simulink model "ML_UAV_3D_2"  (R2018a)
settings: Solver=ode4  StartTime=0.0  StopTime=130  FixedStep=Ts  MaxStep=2*T  MinStep=T  RelTol=1e-4
values from neighbouring files (symbols this model uses):
  Ac = 0.0331    [init_ML_UAV_3D_2.m]
  Am1_LPF = sysd.denominator{1}    [init_ML_UAV_3D_2.m]
  Am2_LPF = sysd.denominator{1}    [init_ML_UAV_3D_2.m]
  Am_coup_LPF = sysd.denominator{1}    [init_ML_UAV_3D_2.m]
  Amp_sf = 3    [init_ML_UAV_3D_2.m]
  Amp_sf_rp = 0.05*uav.m*g    [init_ML_UAV_3D_2.m]
  Bm1_LPF = sysd.numerator{1}    [init_ML_UAV_3D_2.m]
  Bm2_LPF = sysd.numerator{1}    [init_ML_UAV_3D_2.m]
  Bm_coup_LPF = sysd.numerator{1}    [init_ML_UAV_3D_2.m]
  C_S = [5;5;9]*10^-3    [init_ML_UAV_3D_2.m]
  Cd_u = 0.2    [init_ML_UAV_3D_2.m]
  dc_M_p = 6.7    [init_ML_UAV_3D_2.m]
  eps_V = 0.5    [init_ML_UAV_3D_2.m]
  g = 9.81    [init_ML_UAV_3D_2.m]
  gamma_d_p = (2*0.3/0.03*2*0.2*12/4)/10    (= 2.4)    [init_ML_UAV_3D_2.m]
  k3 = 24    [init_ML_UAV_3D_2.m]
  k4 = 0.8    [init_ML_UAV_3D_2.m]
  min_sf = 5    [init_ML_UAV_3D_2.m]
  min_sf_rp = 0.35*uav.m*g    [init_ML_UAV_3D_2.m]
  OMEGA_FILTER_OUTER = 40    [estimation.m]
  T_init = 10    [init_ML_UAV_3D_2.m]
  Tc = 1/500    (= 0.002)    [estimation.m]
  Tg = 1/ 20    (= 0.05)    [estimation.m]
  Tn = 1/500    (= 0.002)    [estimation.m]
  Ts = 1/500    (= 0.002)    [estimation.m]    (also in init_ML_UAV_3D_2.m)
  Tsc = 1/100    (= 0.01)    [estimation.m]
  Tz = 1/500    (= 0.002)    [estimation.m]
  X_GPS_offset = [0.01 0.005]    [estimation.m]
undefined symbols (not defined in the file or in its folder): Am_HPF, Am_LPF, Am_LPF2, an1, an1_v, an2, an3, Bm_HPF, Bm_LPF, Bm_LPF2, bn1, bn1_v, bn2, bn3, buoy, cable, controller, current, D_b, DiscIntNeverNeededParam, F, filters, J_u, K, kd_t, kp_t, L, Light, magnitude, MIL, Phi0, Psi0, R_b, T, Theta0, theta_q_ini, tolerences, torque_corr, uav, Vol_b, water, wave, X0_u
libraries: simulink x48, simulink_extras x10, UAV_Control x4, dspmtrx3 x2, aerolibwind2 x2
(part 2 of 6)

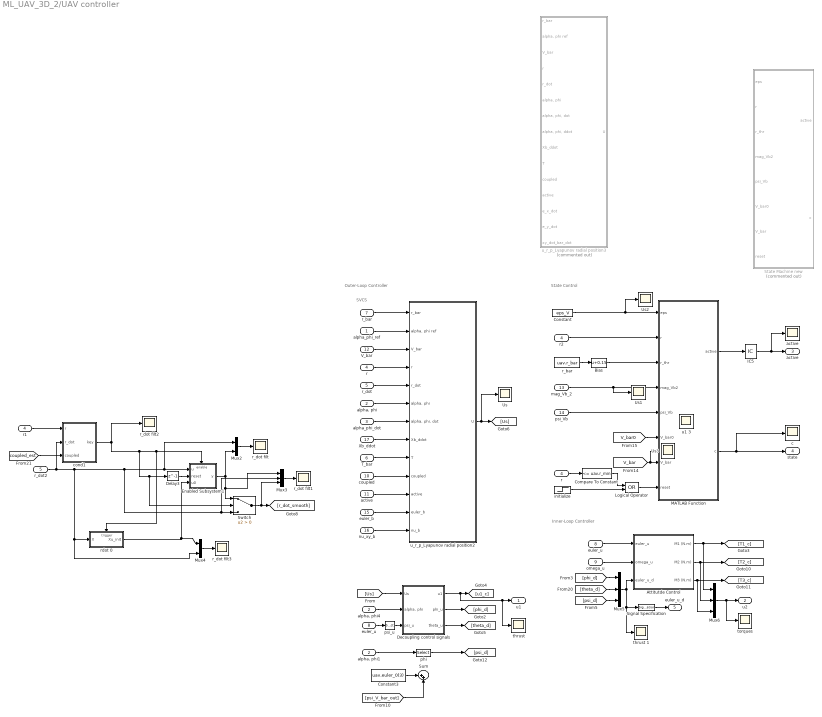
== system ML_UAV_3D_2/UAV controller ==
  note: State Control
  note: Inner-Loop Controller
  note: Outer-Loop Controller
  note: SVCS
  alpha_phi_ref : Inport
  "alpha, phi" : Inport  Port=2
  alpha_phi_dot : Inport  Port=3
  r : Inport  Port=4
  r_dot : Inport  Port=5
  T_bar : Inport  Port=6
  r_bar : Inport  Port=7
  euler_u : Inport  Port=8
  omega_u : Inport  Port=9
  coupled : Inport  Port=10
  active : Inport  Port=11
  V_bar : Inport  Port=12
  mag_Vb_2 : Inport  Port=13
  psi_Vb : Inport  Port=14
  euler_b : Inport  Port=15
  nu_xy_b : Inport  Port=16
  Xb_ddot : Inport  Port=17
  " active " : Scope
  " c " : Scope
  " phi " : Selector  InputPortWidth=2  IndexOptions=Index vector (dialog)  Indices=2  OutputSizes=1
  " r" : InportShadow  Port=4
  " r1" : InportShadow  Port=4
  Attitutde Control : Subsystem
  Bias : Bias  Bias=0.15
  Compare To Constant : simulink/Logic and Bit Operations/Compare To Constant  relop=<=  const=uav.r_min  OutDataTypeStr=boolean
  Constant : Constant  Value=eps_V
  Constant3 : Constant  Value=uav.euler_0(3)
  "Decoupling control signals " : Subsystem
  Delay3 : Delay  DelayLength=1  InitialCondition=0
  Enabled Subsystem1 : Subsystem  TreatAsAtomicUnit=on
  IC5 : InitialCondition  Value=0
  Logical Operator : Logic  Operator=OR  AllPortsSameDT=off  OutDataTypeStr=boolean
  MATLAB Function : MATLAB Function  TreatAsAtomicUnit=on
  Mux2 : Mux  Inputs=2
  Mux3 : Mux  Inputs=3
  Mux4 : Mux  Inputs=2
  Mux5 : Mux  Inputs=3
  Mux6 : Mux  Inputs=3
  Signal Specification : SignalSpecification  Dimensions=[3,1]
  State Machine new : MATLAB Function  Commented=on  TreatAsAtomicUnit=on  SystemSampleTime=Ts  mask{eps_V=0}
  Sum : Sum  Inputs=|++
  Switch : Switch  Criteria=u2 > Threshold
  Us{,1..3} (4 alike) : Scope
  "alpha, phi1" : InportShadow  Port=2
  "alpha, phi4" : InportShadow  Port=2
  cond1 : Subsystem
  "euler_u " : InportShadow  Port=8
  initialize : Step  Time=T_init  Before=1  After=0  SampleTime=0
  psi_u : Selector  InputPortWidth=3  IndexOptions=Index vector (dialog)  Indices=3  OutputSizes=1
  r2 : InportShadow  Port=4
  "r_bar " : Constant  Value=uav.r_bar
  r_dot filt{,1..3} (4 alike) : Scope
  r_dot2 : InportShadow  Port=5
  rdot 0 : Subsystem  TreatAsAtomicUnit=on
  "thrust " : Scope
  thrust 1 : Scope
  torques : Scope
  u1 3 : Scope
  u_r_p_Lyapunov radial position2 : Subsystem
  u_r_p_Lyapunov radial position3 : Subsystem  Commented=on
  u1 : Outport
  u2 : Outport  Port=2
  " active" : Outport  Port=3
  state : Outport  Port=4
  euler_u_d : Outport  Port=5
  wires:
  "Decoupling control signals "/1(u1) -> "thrust "/1, u1/1, [u1_c]
  T_bar/1 -> u_r_p_Lyapunov radial position2/9(T)
  V_bar/1 -> u_r_p_Lyapunov radial position2/3("V_bar ")
  Xb_ddot/1 -> u_r_p_Lyapunov radial position2/8(Xb_ddot)
  alpha_phi_ref/1 -> u_r_p_Lyapunov radial position2/2("alpha, phi ref")
  [V_bar0] -> MATLAB Function/6(V_bar0)
  Constant/1 -> Us2/1, MATLAB Function/1(eps)
  MATLAB Function/1(active) -> IC5/1
  MATLAB Function/2(c) -> " c "/1, state/1
  IC5/1 -> " active "/1, " active"/1
  r_bar/1 -> u_r_p_Lyapunov radial position2/1("r_bar ")
  r/1 -> Compare To Constant/1
  Compare To Constant/1 -> Logical Operator/1
  initialize/1 -> Logical Operator/2
  active/1 -> u_r_p_Lyapunov radial position2/11(active)
  "r_bar "/1 -> Bias/1
  u_r_p_Lyapunov radial position2/1(U) -> Us/1, [Us]
  Logical Operator/1 -> MATLAB Function/8(reset)
  Mux2/1 -> r_dot filt/1
  Enabled Subsystem1/1(y) -> Mux2/2, Mux3/1, Switch/1
  Switch/1 -> Mux3/3, [r_dot_smooth]
  Mux3/1 -> r_dot filt1/1
  [coupled_est] -> cond1/3(coupled)
  coupled/1 -> u_r_p_Lyapunov radial position2/10(coupled)
  r_dot2/1 -> cond1/2(r_dot), Enabled Subsystem1/1(u), Mux2/1, Mux3/2, Switch/3, rdot 0/1(X), Mux4/2
  Mux4/1 -> r_dot filt3/1
  rdot 0/1(Xu_init) -> Mux4/1, Enabled Subsystem1/3(u0)
  " r1"/1 -> cond1/1(r)
  cond1/1(key) -> Delay3/1, Switch/2, rdot 0/Trigger, Enabled Subsystem1/Enable, r_dot filt2/1
  Delay3/1 -> Enabled Subsystem1/2(reset)
  [V_bar] -> Us3/1, MATLAB Function/7(V_bar)
  Bias/1 -> MATLAB Function/3(r_thr)
  r2/1 -> MATLAB Function/2(r)
  "euler_u "/1 -> psi_u/1
  "alpha, phi4"/1 -> "Decoupling control signals "/2("alpha, phi")
  "Decoupling control signals "/3(theta_u) -> [theta_d]
  "Decoupling control signals "/2(phi_u) -> [phi_d]
  euler_u/1 -> Attitutde Control/1(euler_u)
  omega_u/1 -> Attitutde Control/2(omega_u)
  [theta_d] -> Mux5/2
  [phi_d] -> Mux5/1
  [psi_d] -> Mux5/3
  Attitutde Control/1(M1 (N.m)) -> [T1_c], Mux6/1
  Attitutde Control/2(M2 (N.m)) -> [T2_c], Mux6/2
  Attitutde Control/3(M3 (N.m)) -> [T3_c], Mux6/3
  Mux6/1 -> torques/1, u2/1
  "alpha, phi"/1 -> u_r_p_Lyapunov radial position2/6("alpha, phi")
  alpha_phi_dot/1 -> u_r_p_Lyapunov radial position2/7("alpha, phi, dot")
  " r"/1 -> u_r_p_Lyapunov radial position2/4(r)
  r_dot/1 -> u_r_p_Lyapunov radial position2/5(r_dot)
  [Us] -> "Decoupling control signals "/1(Us)
  mag_Vb_2/1 -> Us1/1, MATLAB Function/4(mag_Vb2)
  psi_Vb/1 -> MATLAB Function/5(psi_Vb)
  " phi "/1 -> [psi_d]
  "alpha, phi1"/1 -> " phi "/1
  Mux5/1 -> Signal Specification/1, thrust 1/1, Attitutde Control/3(euler_u_d)
  psi_u/1 -> "Decoupling control signals "/3(psi_u)
  Signal Specification/1 -> euler_u_d/1
  Constant3/1 -> Sum/1
  [psi_V_bar_out] -> Sum/2
  euler_b/1 -> u_r_p_Lyapunov radial position2/12(euler_b)
  nu_xy_b/1 -> u_r_p_Lyapunov radial position2/13(nu_b)

== system ML_UAV_3D_2/Wind model ==
  Bias : Bias  Bias=0.05
  Discrete Wind Gust Model : aerolibwind2/Discrete Wind Gust Model  units=Metric (MKS)  Gx=on  Gy=off  Gz=off  t_0=1  d_m=[1 1 80]  v_m=air.V_wind
      settings: SourceProductName=Aerospace Blockset
  Dryden Wind Turbulence Model (Continuous (+q +r)) : aerolibwind2/Dryden Wind Turbulence Model  (Continuous (+q -r))  Commented=on  units=Metric (MKS)  spec=MIL-F-8785C  model=Continuous Dryden (+q +r)  W20=20  Wdeg=30  TurbProb=10^-2 - Light  L_high=533.4  Wingspan=1.5  ts=0.02  Seed=[11341 23342 13423 13344]  T_on=on
      settings: SourceProductName=Aerospace Blockset
  From25 : From  Commented=on  GotoTag=X_u  TagVisibility=global
  From3 : From  Commented=on  GotoTag=DCM_b2e  TagVisibility=global
  Gain : Gain  Commented=on
  Math Function1 : Math  Commented=on  Operator=transpose  SaturateOnIntegerOverflow=on
  N3 : Scope
  Selector2 : Selector  Commented=on  InputPortWidth=3  IndexOptions=Index vector (dialog)  Indices=2  OutputSizes=1
  Selector6 : Selector  Commented=on  InputPortWidth=2  IndexOptions=Index vector (dialog)  Indices=2  OutputSizes=1
  Zero-Order Hold : ZeroOrderHold  SampleTime=-1
  magnitude : Subsystem
  V_wind : Outport
  omega_wind : Outport  Port=2
  wires:
  Selector6/1 -> Gain/1
  Gain/1 -> Dryden Wind Turbulence Model (Continuous (+q +r))/1
  Bias/1 -> Dryden Wind Turbulence Model (Continuous (+q +r))/2, Discrete Wind Gust Model/1
  Math Function1/1 -> Dryden Wind Turbulence Model (Continuous (+q +r))/3
  From3/1 -> Math Function1/1
  Dryden Wind Turbulence Model (Continuous (+q +r))/2 -> Selector2/1
  magnitude/1(Out1) -> Bias/1
  From25/1 -> Selector6/1
  [Xdot_u] -> magnitude/1(In1)
  Discrete Wind Gust Model/1 -> Zero-Order Hold/1
  Selector2/1 -> omega_wind/1
  Zero-Order Hold/1 -> V_wind/1, N3/1

== system ML_UAV_3D_2/Preprocessing Unit/smooth lower bound1 ==
  u : Inport
  Manual Switch : ManualSwitch
  Mux3 : Mux  Inputs=2
  Saturation1 : Saturate  UpperLimit=inf  LowerLimit=min_sf
  apply for lower bound only : Switch  Criteria=u2 > Threshold  Threshold=Amp_sf+min_sf
  sat : Scope
  saturation function : Fcn  Expr=Amp_sf*tanh((u(1)-(Amp_sf+min_sf))/(Amp_sf)) + (Amp_sf+min_sf)
  sat(u) : Outport
  wires:
  apply for lower bound only/1 -> Manual Switch/1
  Mux3/1 -> sat/1
  saturation function/1 -> Mux3/2, apply for lower bound only/3
  u/1 -> Saturation1/1, apply for lower bound only/1, Mux3/1, apply for lower bound only/2, saturation function/1
  Saturation1/1 -> Manual Switch/2
  Manual Switch/1 -> sat(u)/1

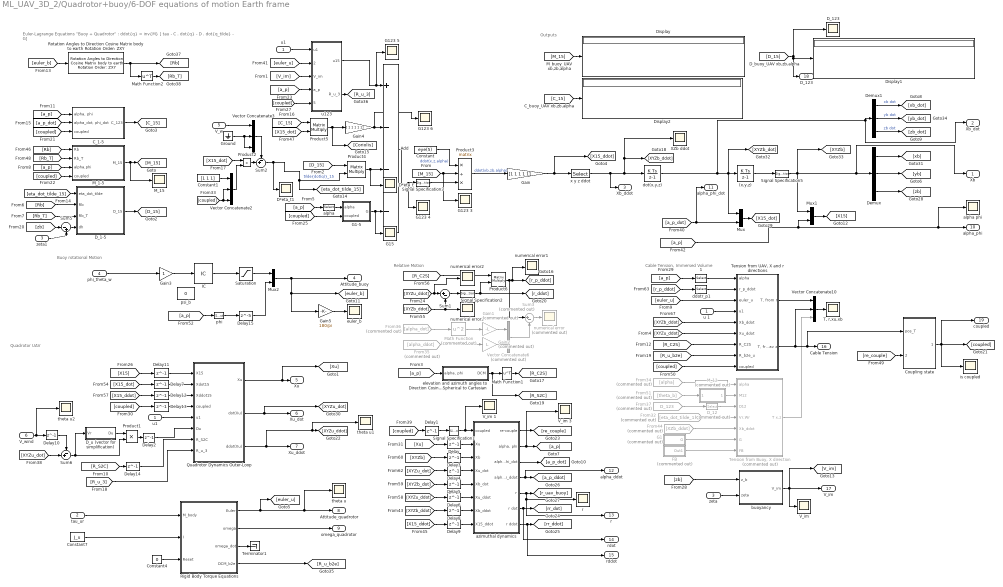
== system ML_UAV_3D_2/Quadrotor+buoy/6-DOF equations of motion Earth frame ==
  note: Relative Motion
  note: Outputs
  note: Buoy rotational Motion
  note: Cable Tension, Immersed Volume
  note: Quadrotor UAV
  note: Euler-Lagrange Equations "Buoy + Quadrotor" : ddot{q} = inv{M} [ tau - C . dot{q} - D . dot{q_tilde} - G]
  u1 : Inport
  tau_ur : Inport  Port=2
  zeta : Inport  Port=3
  phi_theta_w : Inport  Port=4
  V_w : Inport  Port=5
  V_wind : Inport  Port=6
  "  r   " : Scope
  " 1 " : Selector  InputPortWidth=2  IndexOptions=Index vector (dialog)  Indices=1  OutputSizes=2
  " alpha " : Selector  InputPortWidth=2  IndexOptions=Index vector (dialog)  Indices=1  OutputSizes=1
  (x,y,z) : DiscreteIntegrator  InitialCondition=[pos_b_ini]  SampleTime=-1  ICPrevOutput=DiscIntNeverNeededParam  ICPrevScaledInput=DiscIntNeverNeededParam
  Add : Sum  Inputs=+---
  C_1-5 : Subsystem
  Constant : Constant  Value=eye(5)
  Constant1 : Constant  Value=[1 1 1]
  Constant4 : Constant  Value=0
  Constant7 : Constant  Value=J_u
  Coupling state : Subsystem
  D*eta_t : Scope
  D*eta_t1 : Scope
  D_1-5 : Subsystem
  D_12 : Selector  Commented=on  NumberOfDimensions=2  InputPortWidth=3  IndexOptions=Starting index (dialog),Starting index (dialog)  Indices=1,1  OutputSizes=2,2
  "D_123   " : Scope
  D_u (vector for simplification) : Subsystem
  Delay{,3..9,11..14} (12 alike) : Delay  DelayLength=1
  Delay1 : Delay  DelayLength=1  InitialCondition=0
  Delay10 : Delay  DelayLength=1  InitialCondition=[0;0;0]
  Delay15 : Delay  DelayLength=5
  Delay2 : Delay  DelayLength=1  InitialCondition=[0; 0; 0]
  Demux : Demux  Outputs=3
  Demux1 : Demux  Outputs=3
  Display : Display
  Display1 : Display
  Display2 : Display
  FB : Subsystem  Commented=on
  From32 : From  Commented=on  GotoTag=eta_dot_tilde_12
  From34 : From  Commented=on  GotoTag=alpha
  From35 : From  Commented=on  GotoTag=alpha_ddot
  From36 : From  Commented=on  GotoTag=alpha_dot
  From37 : From  Commented=on  GotoTag=D_123
  From44 : From  Commented=on  GotoTag=XZb_ddot
  From51 : From  Commented=on  GotoTag=theta_b
  G1 : Subsystem  Commented=on
  G1-5 : Subsystem
  G123 {3..6} (4 alike) : Scope
  "G15 " : Scope
  Gain : Gain  Gain=[1 1 1 1 1]
  Gain1 : Gain  Commented=on  Gain=-L
  Gain2 : Gain  Commented=on  Gain=L
  Gain3 : Gain
  Gain4 : Gain  Gain=[ 1 1 1 1 1]
  Gain5 : Gain  Gain=180/pi
  Ground : Ground
  IC : InitialCondition  Value=[0 0]
  M_1-5 : Subsystem
  M_12 : Subsystem  Commented=on
  M_15 : Scope
  Math Function : Math  Commented=on  Operator=square  SaturateOnIntegerOverflow=on
  Math Function1 : Math  Operator=transpose  SaturateOnIntegerOverflow=on
  Math Function2 : Math  Operator=transpose  SaturateOnIntegerOverflow=on
  Mux : Mux  Inputs=2
  Mux1 : Mux  Inputs=2
  Mux2 : Mux  Inputs=2
  Product1 : Product  Inputs=**  SaturateOnIntegerOverflow=on  InputSameDT=on  OutDataTypeStr=Inherit: Same as first input
  Product2 : Product  Inputs=**  SaturateOnIntegerOverflow=on  InputSameDT=on  OutDataTypeStr=Inherit: Same as first input
  Product3 : Product  Inputs=*/*  Multiplication=Matrix(*)  SaturateOnIntegerOverflow=on  InputSameDT=on  OutDataTypeStr=Inherit: Same as first input
  Product4 : Product  Inputs=**  Multiplication=Matrix(*)  SaturateOnIntegerOverflow=on  InputSameDT=on  OutDataTypeStr=Inherit: Same as first input
  Product5 : Product  Inputs=**  Multiplication=Matrix(*)  SaturateOnIntegerOverflow=on  InputSameDT=on  OutDataTypeStr=Inherit: Same as first input
  Product6 : Product  Multiplication=Matrix(*)
  Quadrotor Dynamics Outer-Loop : Subsystem
  "Rigid Body Torque Equations " : Subsystem  AncestorBlock=UAV_Control/Rigid Body Torque Equations  mask(Rotational motion of rigid body){euler0=euler_u_ini, omega0=omega_u_ini}
      mask prompts: euler0 "Initial euler angles:"; omega0 "Initial angular velocites:"
      mask help: Determines the rotational motion of a 6DOF rigid body.
      mask Help:
      | alpha=Mb/I - omega x (I.omega)
      | omega_dot=alpha
      | 
      | Euler_dot=R x omega
      mask Display:
      | port_label('input',1,'M_b (N.m)','texmode','on')
      | port_label('input',2,'I (kg/m^2)','texmode','on')
      | port_label('input',3,'Reset','texmode','on')
      | 
      | port_label('output',1,'\phi,\theta,\psi (rad)','texmode','on')
      | port_label('output',2,'\omega (rad/s)','texmode','on')
      | port_label('output',3,'\alpha (rad/s^2)','texmode','on')
      | port_label('output',4,'DCM_{b2e}','texmode','on')
  Rotation Angles to Direction Cosine Matrix body to earth Rotation Order: ZXY : UAV_Control/Rotation Angles to Direction Cosine Matrix body to earth Rotation Order: ZXY
      settings: SourceProductName=UAV_Control
  Saturation : Saturate  UpperLimit=[0.15 0.15]  LowerLimit=[-0.15 -0.15]
  Signal Specification1 : SignalSpecification  Dimensions=1
  Signal Specification2 : SignalSpecification  Dimensions=3
  Signal Specification3 : SignalSpecification  Dimensions=5
  Signal Specification5 : SignalSpecification  Dimensions=3
  Sum1 : Sum  Inputs=|+-
  Sum2 : Sum  Inputs=-+|  SaturateOnIntegerOverflow=on
  Sum3 : Sum  Commented=on  Inputs=|+-
  Sum5 : Sum  Inputs=|-+  SaturateOnIntegerOverflow=on
  Sum6 : Sum  Inputs=-+|  SaturateOnIntegerOverflow=on
  "T, r,xu,xb" : Scope
  "Tension from Buoy, X direction" : Subsystem  Commented=on
  "Tension from UAV, X and r directions" : Subsystem
  Terminator1 : Terminator
  "V_im " : Scope
  V_im 1 : Scope
  V_im 3 : Scope
  Vector Concatenate10 : Concatenate  NumInputs=3
  Vector Concatenate2 : Concatenate  NumInputs=3
  Vector Concatenate3 : Concatenate  NumInputs=3
  Vector Concatenate6 : Concatenate  Commented=on
  "XZb ddot " : Scope
  "alpha phi   " : Scope
  azimuthal dynamics : Subsystem
  buoyancy : Subsystem
  ddotr_p1 : Selector  InputPortWidth=3  IndexOptions=Index vector (dialog)  Indices=1  OutputSizes=2
  dot(x,y,z) : DiscreteIntegrator  InitialCondition=[v_b_ini]  SampleTime=-1  ICPrevOutput=DiscIntNeverNeededParam  ICPrevScaledInput=DiscIntNeverNeededParam
  elevation and azimuth angles to Direction Cosine Matrix Spherical to Cartesian : Subsystem
      mask Display:
      | port_label('input',1,'\alpha, \phi','texmode','on')
      | port_label('output',1,'DCM_{S2C}','texmode','on')
  euler_b : Scope
  "is coupled " : Scope
  numerical error : Scope  Commented=on
  numerical error1 : Scope
  numerical error2 : Scope
  numerical error3 : Scope
  "phi  " : Selector  InputPortWidth=2  IndexOptions=Index vector (dialog)  Indices=2  OutputSizes=1
  psi_b : Constant  Value=0
  theta u : Scope
  theta u1 : Scope
  theta u2 : Scope
  u 1 : InportShadow
  "u1  " : InportShadow
  u123 : Subsystem
  x y z ddot : Selector  InputPortWidth=5  IndexOptions=Index vector (dialog)  Indices=[1 2 3]  OutputSizes=1
  zeta1 : InportShadow  Port=3
  Xb : Outport  Unit=m  InitialOutput=0
  Xb_dot : Outport  Port=2  Unit=m  InitialOutput=0
  Xb_ddot : Outport  Port=3  Unit=m  InitialOutput=0
  Attitude_buoy : Outport  Port=4  Unit=rad/s^2  InitialOutput=0
  Xu : Outport  Port=5  Unit=m  InitialOutput=0
  Xu_dot : Outport  Port=6  Unit=m/s  InitialOutput=0
  Xu_ddot : Outport  Port=7  Unit=m/s  InitialOutput=0
  Attitude_quadrotor : Outport  Port=8  Unit=rad  InitialOutput=0
  omega_quadrotor : Outport  Port=9  Unit=rad/s  InitialOutput=0
  alpha_phi : Outport  Port=10  Unit=m  InitialOutput=0
  alpha_phi_dot : Outport  Port=11  Unit=m  InitialOutput=0
  alpha_ddot : Outport  Port=12  Unit=m  InitialOutput=0
  "  r" : Outport  Port=13  Unit=m  InitialOutput=0
  "  rdot" : Outport  Port=14  Unit=m  InitialOutput=0
  "  rddot" : Outport  Port=15  Unit=m  InitialOutput=0
  Cable Tension : Outport  Port=16  Unit=rad/s^2  InitialOutput=0
  V_im : Outport  Port=17  Unit=m  InitialOutput=0
  "D_123 " : Outport  Port=18  Unit=m  InitialOutput=0
  coupled : Outport  Port=19  Unit=m  InitialOutput=0
  wires:
  u123/1(u15) -> G123 5/1, Add/1
  Product4/1 -> D*eta_t/1, Add/3
  [D_15] -> Product4/1
  Sum2/1 -> D*eta_t1/1, [eta_dot_tilde_15], Product4/2  "tilde{dot(q)}_15"
  G1-5/1(G) -> "G15 "/1, Add/4
  [a_p] -> Mux1/2, "alpha phi   "/1, alpha_phi/1
  [Rb] -> D_1-5/2(Rb)
  D_1-5/1(D_15) -> [D_15]
  [Rb] -> M_1-5/1(Rb)
  [a_p] -> M_1-5/3(alpha,phi)
  Demux1/3 -> [zb_dot]  "zb dot"
  Demux1/1 -> [xb_dot]  "xb dot"
  Vector Concatenate3/1 -> Sum2/1
  phi_theta_w/1 -> Gain3/1
  "Rigid Body Torque Equations "/1("Euler ") -> [euler_u], theta u/1, Attitude_quadrotor/1
  Constant7/1 -> "Rigid Body Torque Equations "/2(I)
  tau_ur/1 -> "Rigid Body Torque Equations "/1(M_body)
  [euler_u] -> u123/2(euler_u)
  [V_im] -> u123/3(V_im)
  [a_p] -> " alpha "/1
  Demux/1 -> [xb]
  Demux/2 -> [yb]
  M_1-5/1(M_15) -> M_15/1, [M_15]
  [M_15] -> G123 3/1, Product3/2
  Constant/1 -> Product3/1  "ddot(x,z,alpha)"
  Product3/1 -> Gain/1  "ddot(xb,zb,alpha)"
  IC/1 -> Saturation/1
  [a_p] -> C_1-5/1("alpha, phi ")
  [a_p_dot] -> C_1-5/2("alpha_dot, phi_dot")
  C_1-5/1(C_123) -> [C_15]
  [C_15] -> Product5/1
  Product5/1 -> [Coriolis], Gain4/1
  Gain/1 -> [X15_ddot], x y z ddot/1
  [a_p] -> u123/4(a_p)
  [r_p_ddot] -> ddotr_p1/1
  [euler_u] -> "Tension from UAV, X and r directions"/3(euler_u)
  u 1/1 -> "Tension from UAV, X and r directions"/4(u1)
  [D_15] -> Display1/1, "D_123 "/1, "D_123   "/1
  [M_15] -> Display/1
  [C_15] -> Display2/1
  (x,y,z)/1 -> Signal Specification5/1
  [zb] -> buoyancy/1(z_b)
  zeta/1 -> buoyancy/2(zeta)
  From34/1 -> "Tension from Buoy, X direction"/1(alpha)
  D_12/1 -> "Tension from Buoy, X direction"/3(D12)
  buoyancy/1(V_im) -> "V_im "/1, V_im/1, [V_im]
  M_12/1(M_12) -> "Tension from Buoy, X direction"/2(M12)
  From37/1 -> D_12/1
  From44/1 -> "Tension from Buoy, X direction"/5(Xb_ddot)
  From32/1 -> "Tension from Buoy, X direction"/4(Vr,Wr)
  [XYZb_ddot] -> "Tension from UAV, X and r directions"/5(Xb_ddot)
  G1/1(G) -> "Tension from Buoy, X direction"/6(G)
  From51/1 -> M_12/1(theta)
  x y z ddot/1 -> Xb_ddot/1, [XYZb_ddot], "XZb ddot "/1, dot(x,y,z)/1
  ddotr_p1/1 -> "Tension from UAV, X and r directions"/2(r_p_ddot)
  [XYZu_ddot] -> "Tension from UAV, X and r directions"/6(Xu_ddot)
  FB/1(Out1) -> "Tension from Buoy, X direction"/7(FB)
  Vector Concatenate10/1 -> "T, r,xu,xb"/1
  "Tension from Buoy, X direction"/1(T x,z) -> Vector Concatenate10/3
  Gain2/1 -> Vector Concatenate6/2
  [R_C2S] -> Product6/1
  Vector Concatenate6/1 -> Sum3/2
  elevation and azimuth angles to Direction Cosine Matrix Spherical to Cartesian/1(DCM) -> [R_S2C], Math Function1/1
  Product6/1 -> Sum3/1, numerical error1/1, [r_p_ddot]
  Gain1/1 -> Vector Concatenate6/1
  Math Function/1 -> Gain1/1
  Sum1/1 -> Signal Specification2/1
  [XYZu_ddot] -> numerical error2/1, Sum1/1
  Math Function1/1 -> [R_C2S]
  Sum3/1 -> numerical error/1
  [XYZb_ddot] -> numerical error3/1, Sum1/2
  From36/1 -> Math Function/1
  Mux2/1 -> Gain5/1, [euler_b], Attitude_buoy/1
  Add/1 -> Signal Specification3/1, G123 4/1
  Gain3/1 -> IC/1
  Gain4/1 -> Add/2, G123 6/1
  [eta_dot_tilde_15] -> D_1-5/1(eta_dot_tilde)
  Sum5/1 -> D_1-5/4(dh)
  [zb] -> Sum5/1
  zeta1/1 -> Sum5/2
  [coupled] -> C_1-5/3(coupled)
  [coupled] -> M_1-5/4(coupled)
  [coupled] -> G1-5/2(coupled)
  u1/1 -> u123/1(u1)
  [X15_dot] -> Product5/2
  Signal Specification2/1 -> Product6/2, [r_ddot]
  Signal Specification3/1 -> Product3/3
  Quadrotor Dynamics Outer-Loop/1(Xu) -> [Xu], Xu/1
  [coupled] -> Delay13/1
  "u1  "/1 -> Quadrotor Dynamics Outer-Loop/5(u1)
  Quadrotor Dynamics Outer-Loop/2(dot(Xu)) -> [XYZu_dot], Xu_dot/1
  [coupled] -> u123/5(coupled)
  Vector Concatenate2/1 -> Product2/2
  [Xu] -> Delay/1
  azimuthal dynamics/1(re-couple) -> [re_couple]
  azimuthal dynamics/2("alpha, phi") -> V_im 3/1, [a_p]
  azimuthal dynamics/3("alpha_dot, phi_dot ") -> [a_p_dot]
  azimuthal dynamics/4("alpha_ddot, phi_ddot") -> alpha_ddot/1, [a_p_ddot]
  Delay/1 -> azimuthal dynamics/2(Xu)
  azimuthal dynamics/5("r ") -> "  r"/1, "  r   "/1, [r_uav_buoy]
  [X15] -> Delay11/1
  Delay3/1 -> azimuthal dynamics/3(Xb)
  [X15_ddot] -> Delay12/1
  [X15_dot] -> Delay7/1
  dot(x,y,z)/1 -> Mux/1, (x,y,z)/1, [XYZb_dot], Xb_dot/1, Demux1/1
  [a_p_dot] -> alpha_phi_dot/1, Mux/2
  Mux/1 -> [X15_dot]
  Mux1/1 -> [X15]
  Signal Specification5/1 -> [XYZb], Mux1/1, Xb/1, Demux/1
  [a_p] -> " 1 "/1
  [XYZb] -> Delay3/1
  [XYZu_dot] -> Delay4/1
  [XYZb_dot] -> Delay5/1
  [XYZu_ddot] -> Delay6/1
  [XYZb_ddot] -> Delay8/1
  From35/1 -> Gain2/1
  Delay4/1 -> azimuthal dynamics/4("Xu_dot ")
  [X15_ddot] -> Delay9/1
  Delay5/1 -> azimuthal dynamics/5(Xb_dot)
  Delay6/1 -> azimuthal dynamics/6(Xu_ddot)
  Delay8/1 -> azimuthal dynamics/7("Xb_ddot   ")
  Delay9/1 -> azimuthal dynamics/8("X15_ddot  ")
  [coupled] -> Delay1/1
  Delay11/1 -> Quadrotor Dynamics Outer-Loop/1(X15)
  Delay12/1 -> Quadrotor Dynamics Outer-Loop/3(Xddot15)
  Delay7/1 -> Quadrotor Dynamics Outer-Loop/2(Xdot15)
  Delay13/1 -> Quadrotor Dynamics Outer-Loop/4(coupled)
  azimuthal dynamics/6(r dot) -> "  rdot"/1, [rr_dot]
  azimuthal dynamics/7(r ddot) -> "  rddot"/1, [rr_ddot]
  "Tension from UAV, X and r directions"/2("T, from uav z") -> Vector Concatenate10/2, Coupling state/1(pos_T), Cable Tension/1
  [re_couple] -> Coupling state/2(re_couple)
  Coupling state/1(is coupled) -> "is coupled "/1, coupled/1, [coupled]
  Quadrotor Dynamics Outer-Loop/3(ddot(Xu)) -> Xu_ddot/1, theta u1/1, [XYZu_ddot]
  "Tension from UAV, X and r directions"/1("T, from r") -> Vector Concatenate10/1
  D_u (vector for simplification)/1(Du) -> Product1/1
  [XYZu_dot] -> Sum6/2
  Sum6/1 -> D_u (vector for simplification)/1(Vr), Product1/2
  Ground/1 -> Vector Concatenate3/3, Vector Concatenate3/2
  V_w/1 -> Vector Concatenate3/1
  Product2/1 -> Sum2/2
  [X15_dot] -> Product2/1
  [coupled] -> Vector Concatenate2/2, Vector Concatenate2/3
  Constant1/1 -> Vector Concatenate2/1
  " alpha "/1 -> G1-5/1(alpha)
  Demux1/2 -> [yb_dot]  "yb dot"
  Demux/3 -> [zb]
  Gain5/1 -> euler_b/1
  [a_p] -> elevation and azimuth angles to Direction Cosine Matrix Spherical to Cartesian/1("alpha, phi")
  [R_C2S] -> "Tension from UAV, X and r directions"/7(R_C2S)
  Constant4/1 -> "Rigid Body Torque Equations "/3(Reset)
  "Rigid Body Torque Equations "/2(omega) -> omega_quadrotor/1
  "Rigid Body Torque Equations "/4(DCM_b2e) -> [R_u_b2e]
  "Rigid Body Torque Equations "/3(omega_dot) -> Terminator1/1
  [a_p] -> "phi  "/1
  Saturation/1 -> Mux2/1
  [R_S2C] -> Delay14/1
  Delay14/1 -> Quadrotor Dynamics Outer-Loop/7(R_S2C)
  u123/2(R_u_3) -> [R_u_3]
  [R_u_3] -> Quadrotor Dynamics Outer-Loop/8(R_u_3)
  [R_u_b2e] -> "Tension from UAV, X and r directions"/8("R_b2e_u ")
  " 1 "/1 -> "Tension from UAV, X and r directions"/1(alpha)
  [euler_b] -> Rotation Angles to Direction Cosine Matrix body to earth Rotation Order: ZXY/1
  Rotation Angles to Direction Cosine Matrix body to earth Rotation Order: ZXY/1 -> Math Function2/1, [Rb]
  Math Function2/1 -> [Rb_T]
  [Rb_T] -> M_1-5/2(Rb_T)
  [Rb_T] -> D_1-5/3(Rb_T)
  [coupled] -> "Tension from UAV, X and r directions"/9(coupled)
  Delay10/1 -> Sum6/1
  V_wind/1 -> Delay10/1, theta u2/1
  Product1/1 -> Delay2/1
  Delay2/1 -> Quadrotor Dynamics Outer-Loop/6(Du)
  Delay1/1 -> Signal Specification1/1
  Signal Specification1/1 -> V_im 1/1, azimuthal dynamics/1(coupled)
  "phi  "/1 -> Delay15/1
  Delay15/1 -> Mux2/2

== system ML_UAV_3D_2/Save to file/mean absolute error ==
  In1 : Inport
  Abs : Abs
  Add : Sum
  Constant : Constant  Value=T
  Delay : Delay  DelayLength=1
  IC : InitialCondition
  Product1 : Product  Inputs=*/
  Product2 : Product  Inputs=*/
  Out1 : Outport
  wires:
  Product2/1 -> IC/1
  Add/1 -> Product1/1, Delay/1
  Delay/1 -> Add/1
  [time] -> Product2/1
  In1/1 -> Abs/1
  Product1/1 -> Out1/1
  Constant/1 -> Product2/2
  IC/1 -> Product1/2
  Abs/1 -> Add/2

== system ML_UAV_3D_2/Scope/absolute mean ==
  u : Inport
  Abs : Abs
  Bias : Bias  Bias=1/1000
  Clock : Clock
  Current velocity : Scope
  Current velocity1 : Scope
  Current velocity2 : Scope
  Discrete-Time Integrator : DiscreteIntegrator  gainval=1  SampleTime=Ts  ICPrevOutput=DiscIntNeverNeededParam  ICPrevScaledInput=DiscIntNeverNeededParam
  Divide1 : Product  Inputs=*/
  mean : Outport
  wires:
  Discrete-Time Integrator/1 -> Current velocity1/1, Divide1/1
  Abs/1 -> Discrete-Time Integrator/1
  u/1 -> Current velocity/1, Abs/1
  Divide1/1 -> mean/1
  Clock/1 -> Bias/1
  Bias/1 -> Current velocity2/1, Divide1/2

== system ML_UAV_3D_2/Scope/absolute mean1 ==
  u : Inport
  Abs : Abs
  Bias : Bias  Bias=1/1000
  Clock : Clock
  Current velocity : Scope
  Current velocity1 : Scope
  Current velocity2 : Scope
  Discrete-Time Integrator : DiscreteIntegrator  gainval=1  SampleTime=Ts  ICPrevOutput=DiscIntNeverNeededParam  ICPrevScaledInput=DiscIntNeverNeededParam
  Divide1 : Product  Inputs=*/
  mean : Outport
  wires:
  Clock/1 -> Bias/1
  Divide1/1 -> mean/1
  u/1 -> Abs/1, Current velocity/1
  Abs/1 -> Discrete-Time Integrator/1
  Discrete-Time Integrator/1 -> Divide1/1, Current velocity1/1
  Bias/1 -> Divide1/2, Current velocity2/1

== system ML_UAV_3D_2/Sensors and Filters/Coupling detection by r ==
  In1 : Inport
  In2 : Inport  Port=2
  Constant1 : Constant  Value=0
  Coupling state : Subsystem
  Data Type Conversion : DataTypeConversion  OutDataTypeStr=double
  IC2 : InitialCondition  Value=0
  Switch14 : Switch  Criteria=u2 > Threshold  Threshold=0.5
  cable length with safety margine : simulink/Logic and Bit Operations/Compare To Constant  relop=>=  const=cable.L_0+0.005  OutDataTypeStr=boolean
  is coupled {,2..4} (4 alike) : Scope
  is coupled : Outport
  wires:
  IC2/1 -> Switch14/3
  In1/1 -> is coupled 3/1, Coupling state/1(r_est), is coupled 2/1, cable length with safety margine/1
  Switch14/1 -> [re_couple]
  cable length with safety margine/1 -> is coupled 4/1, Data Type Conversion/1
  [re_couple] -> Coupling state/2(re_couple)
  Data Type Conversion/1 -> IC2/1
  Coupling state/1(is coupled) -> is coupled/1, "is coupled "/1
  Constant1/1 -> Switch14/1
  In2/1 -> Switch14/2

== system ML_UAV_3D_2/Sensors and Filters/Data processing ==
  Acc : Inport
  "GPS " : Inport  Port=2
  p,q,r : Inport  Port=3
  Sonar : Inport  Port=4
  Estimate Attitude : Subsystem  TreatAsAtomicUnit=on  SystemSampleTime=Tc
  Estimate Position : Subsystem  TreatAsAtomicUnit=on  SystemSampleTime=Tc
  "Euler " : Selector  InputPortWidth=5  IndexOptions=Index vector (dialog)  Indices=[3]  OutputSizes=1
  GPS : InportShadow  Port=2
  Xe_est : Outport
  Ve_est : Outport  Port=2
  q_gyro : Outport  Port=3
  "q_est " : Outport  Port=4
  pitch_est : Outport  Port=5
  wires:
  GPS/1 -> "Euler "/1
  Acc/1 -> Estimate Attitude/1(Acc)
  p,q,r/1 -> Estimate Attitude/2(q)
  "Euler "/1 -> Estimate Attitude/3(Euler)
  Estimate Attitude/2(q_f) -> "q_est "/1
  "GPS "/1 -> Estimate Position/1(OptiTrack)
  Estimate Position/1(Xe) -> Xe_est/1
  Estimate Position/2(Ve) -> Ve_est/1
  Estimate Attitude/1(q_g) -> q_gyro/1
  Sonar/1 -> Estimate Position/3(Sonar)
  Estimate Attitude/3(" pitch") -> Estimate Position/2("pitch, Kalman"), pitch_est/1

== system ML_UAV_3D_2/Sensors and Filters/GPS//INS ==
  X : Inport
  X_dot : Inport  Port=2
  X_ddot : Inport  Port=3
  q : Inport  Port=4
  theta : Inport  Port=5
  Discrete Derivative1 : simulink/Discrete/Discrete Derivative  gainval=1.0  ICPrevScaledInput=0.0  OutMin=[]  OutMax=[]  OutDataType=fixdt(1, 16)  OutScaling=2^-10  DoSatur=off
  Discrete Derivative2 : simulink/Discrete/Discrete Derivative  gainval=1.0  ICPrevScaledInput=0.0  OutMin=[]  OutMax=[]  OutDataType=fixdt(1, 16)  OutScaling=2^-10  DoSatur=off
  GPS noise : RandomNumber  Variance=5/10000  Seed=123  SampleTime=Tg
  Gain : Gain  Gain=0.25
  Gain1 : Gain  Gain=0.5
  Gain2 : Gain
  Gain3 : Gain
  Gain4 : Gain
  IMU noise : RandomNumber  Variance=1/10000  Seed=2235  SampleTime=Ts
  Low Pass Filter{1,3..5} (4 alike) : DiscreteTransferFcn  Numerator=filters.Bm_LPF2  Denominator=filters.Am_LPF2
  Low Pass Filter2 : DiscreteTransferFcn  Numerator=filters.Bm_LPF  Denominator=filters.Am_LPF
  Mux4 : Mux  Inputs=3
  Rate Transition : RateTransition
  Rate Transition1 : RateTransition
  Sum{1,3..6} (5 alike) : Sum  Inputs=++|
  q1 : Scope
  q2 : Scope
  q3 : Scope
  X_est : Outport
  X_dot_est : Outport  Port=2
  q_est : Outport  Port=3
  theta_est : Outport  Port=4
  X_ddot_est : Outport  Port=5
  wires:
  Sum4/1 -> X_dot_est/1
  Low Pass Filter1/1 -> Low Pass Filter3/1
  Gain3/1 -> Sum6/1
  q/1 -> Sum6/2
  theta/1 -> Sum5/2
  Gain2/1 -> Sum5/1
  Rate Transition1/1 -> Low Pass Filter2/1
  IMU noise/1 -> Rate Transition1/1
  Mux4/1 -> Gain1/1
  X/1 -> Sum3/2
  GPS noise/1 -> Rate Transition/1
  Rate Transition/1 -> Low Pass Filter1/1
  Sum5/1 -> theta_est/1
  X_dot/1 -> Sum4/2
  Sum3/1 -> X_est/1
  Sum6/1 -> q_est/1
  Low Pass Filter2/1 -> Gain3/1, Gain2/1, q2/1
  Low Pass Filter3/1 -> Mux4/3, Mux4/2, Mux4/1
  Discrete Derivative1/1 -> Low Pass Filter4/1
  Gain1/1 -> Discrete Derivative1/1, Sum3/1, q1/1
  Gain/1 -> Discrete Derivative2/1, Sum4/1, q3/1
  Discrete Derivative2/1 -> Low Pass Filter5/1
  X_ddot/1 -> Sum1/2
  Gain4/1 -> Sum1/1
  Sum1/1 -> X_ddot_est/1
  Low Pass Filter4/1 -> Gain/1
  Low Pass Filter5/1 -> Gain4/1

== system ML_UAV_3D_2/Sensors and Filters/Sensors ==
  note: Gyro noise destroys the estimation
  note: Acc noise does not affect estimation
  "q " : Inport
  Ab : Inport  Port=2
  Xe : Inport  Port=3
  Euler : Inport  Port=4
  " Sonar (10Hz) (true elevation instead real sonar signal)" : Subsystem
  Accelerometer (500Hz) : Subsystem  TreatAsAtomicUnit=on  SystemSampleTime=Ts
  "GPS (10Hz) " : Subsystem  TreatAsAtomicUnit=on  SystemSampleTime=Tg
  Gyro (500Hz) : Subsystem  TreatAsAtomicUnit=on  SystemSampleTime=Ts
  RT : RateTransition  OutPortSampleTime=Ts
  Rate Transition : RateTransition
  Rate Transition1 : RateTransition
  Rate Transition2 : RateTransition  Deterministic=off  InitialCondition=[X0_u Theta0 1 1]
  Z : Selector  InputPortWidth=5  IndexOptions=Index vector (dialog)  Indices=2  OutputSizes=1
  acc : Scope  Commented=on
  pqr : Scope  Commented=on
  rotation matrix R : Subsystem
  Acc : Outport
  GPS : Outport  Port=2
  " q" : Outport  Port=3
  Sonar : Outport  Port=4
  wires:
  Xe/1 -> "GPS (10Hz) "/1(Xe)
  Ab/1 -> RT/1
  "q "/1 -> Gyro (500Hz)/1(q)
  Euler/1 -> rotation matrix R/1(angle (rad)), "GPS (10Hz) "/2(Euler)
  Accelerometer (500Hz)/1(Acc) -> Rate Transition1/1
  Gyro (500Hz)/1(" q") -> Rate Transition/1
  Z/1 -> " Sonar (10Hz) (true elevation instead real sonar signal)"/1(sonar (m))
  " Sonar (10Hz) (true elevation instead real sonar signal)"/1(calib sonar (m)) -> Sonar/1
  Rate Transition/1 -> pqr/1, " q"/1
  Rate Transition1/1 -> acc/1, Acc/1
  RT/1 -> Accelerometer (500Hz)/1(Ab)
  rotation matrix R/1(R) -> "GPS (10Hz) "/3(DCM_b2e)
  Rate Transition2/1 -> Z/1, GPS/1
  "GPS (10Hz) "/1(GPS) -> Rate Transition2/1

== system ML_UAV_3D_2/Sensors and Filters/Sterio camera + encoder ==
  note: the error in alpha should relate to the stereo camera accuracy and the radial distance:
      | alpha = atan( 2cm / 7 m) = 0.0029 rad.
  "alpha, phi" : Inport
  alpha_phi_dot : Inport  Port=2
  alpha_phi_ddot : Inport  Port=3
  r : Inport  Port=4
  r_dot : Inport  Port=5
  r_ddot : Inport  Port=6
  Discrete Derivative{,1..3} (4 alike) : simulink/Discrete/Discrete Derivative  gainval=1.0  ICPrevScaledInput=0.0  OutMin=[]  OutMax=[]  OutDataType=fixdt(1, 16)  OutScaling=2^-10  DoSatur=off
  Gain1 : Gain  Gain=0.5
  Gain2 : Gain  Gain=0.3
  Gain4 : Gain
  Gain5 : Gain
  Gain6 : Gain  Gain=0.25
  Gain7 : Gain  Gain=0.5
  Low Pass Filter{1..9} (9 alike) : DiscreteTransferFcn  Numerator=filters.Bm_LPF2  Denominator=filters.Am_LPF2
  Low Pass Filter10 : DiscreteTransferFcn  Commented=on  Numerator=Bm_LPF2  Denominator=Am_LPF2
  Low Pass Filter11 : DiscreteTransferFcn  Commented=on  Numerator=filters.Bm_LPF2  Denominator=filters.Am_LPF2
  Rate Transition1 : RateTransition
  Rate Transition2 : RateTransition
  Sum{1..2,7..10} (6 alike) : Sum  Inputs=++|
  stereo cam noise (location in frame) : RandomNumber  Variance=1/100000  Seed=5684  SampleTime=Tsc
  sterio cam noise (range) : RandomNumber  Variance=1/1000  Seed=1142  SampleTime=Tsc
  alpha_phi_est : Outport
  alpha_phi_dot_est : Outport  Port=2
  r_est : Outport  Port=3
  r_dot_est : Outport  Port=4
  alpha_phi_ddot_est : Outport  Port=5
  r_ddot_est : Outport  Port=6
  wires:
  Rate Transition2/1 -> Low Pass Filter3/1
  stereo cam noise (location in frame)/1 -> Rate Transition2/1
  Gain5/1 -> Sum8/1
  Sum10/1 -> r_dot_est/1
  Discrete Derivative/1 -> Low Pass Filter8/1
  alpha_phi_dot/1 -> Sum9/2
  Gain4/1 -> Sum7/1
  Discrete Derivative1/1 -> Low Pass Filter7/1
  Sum7/1 -> alpha_phi_est/1
  Sum8/1 -> r_est/1
  r/1 -> Sum8/2
  "alpha, phi"/1 -> Sum7/2
  r_dot/1 -> Sum10/2
  Sum9/1 -> alpha_phi_dot_est/1
  sterio cam noise (range)/1 -> Rate Transition1/1
  Rate Transition1/1 -> Low Pass Filter1/1
  Sum1/1 -> alpha_phi_ddot_est/1
  Discrete Derivative2/1 -> Low Pass Filter6/1
  Gain6/1 -> Discrete Derivative2/1, Sum9/1
  Gain1/1 -> Sum1/1
  alpha_phi_ddot/1 -> Sum1/2
  r_ddot/1 -> Sum2/2
  Discrete Derivative3/1 -> Low Pass Filter9/1
  Gain2/1 -> Sum2/1
  Sum2/1 -> r_ddot_est/1
  Gain7/1 -> Discrete Derivative3/1, Sum10/1
  Low Pass Filter2/1 -> Gain7/1
  Low Pass Filter4/1 -> Gain2/1
  Low Pass Filter5/1 -> Gain6/1
  Low Pass Filter6/1 -> Gain1/1
  Low Pass Filter7/1 -> Low Pass Filter5/1
  Low Pass Filter8/1 -> Low Pass Filter2/1
  Low Pass Filter9/1 -> Low Pass Filter4/1
  Low Pass Filter3/1 -> Gain4/1, Discrete Derivative1/1
  Low Pass Filter1/1 -> Gain5/1, Discrete Derivative/1

== system ML_UAV_3D_2/Sensors and Filters/quadrotor position from relative buoy-UAV position ==
  X_u : Inport
  Xdot_u : Inport  Port=2
  Xddot_u : Inport  Port=3
  r : Inport  Port=4
  r_dot : Inport  Port=5
  r_ddot : Inport  Port=6
  "alpha, phi" : Inport  Port=7
  "(alpha, phi)_dot" : Inport  Port=8
  "(alpha, phi)_ddot" : Inport  Port=9
  Buoy's States from UAV : MATLAB Function  TreatAsAtomicUnit=on
  Demux : Demux  Outputs=2
  Demux3 : Demux  Outputs=2
  Demux4 : Demux  Outputs=2
  Signal Specification{,1..8} (9 alike) : SignalSpecification  Dimensions=[3,1]
  UAV's Spherical States : MATLAB Function  TreatAsAtomicUnit=on
  theta u1 : Scope
  theta u4 : Scope
  theta u6 : Scope
  Xb : Outport
  Xdot_b : Outport  Port=2
  Xddot_b : Outport  Port=3
  wires:
  r/1 -> UAV's Spherical States/1(r)
  Xdot_u/1 -> Signal Specification5/1
  X_u/1 -> Signal Specification/1
  r_dot/1 -> UAV's Spherical States/2(r_dot)
  Buoy's States from UAV/3(rb_ddot) -> Signal Specification3/1
  Buoy's States from UAV/1(rb) -> Signal Specification1/1
  r_ddot/1 -> UAV's Spherical States/3(r_ddot)
  Xddot_u/1 -> Signal Specification2/1
  Demux/1 -> UAV's Spherical States/4(alpha)
  Demux/2 -> UAV's Spherical States/7(phi)
  "alpha, phi"/1 -> Demux/1  "alpha"
  "(alpha, phi)_dot"/1 -> Demux3/1
  Demux3/1 -> UAV's Spherical States/5(alpha_dot)
  Demux4/1 -> UAV's Spherical States/6(alpha_ddot)
  "(alpha, phi)_ddot"/1 -> Demux4/1
  Demux3/2 -> UAV's Spherical States/8(phi_dot)
  Demux4/2 -> UAV's Spherical States/9(phi_ddot)
  UAV's Spherical States/4(R_S2C) -> Buoy's States from UAV/4(R_S2C)
  UAV's Spherical States/2(br_dot) -> Signal Specification7/1
  UAV's Spherical States/1(br) -> Signal Specification6/1
  UAV's Spherical States/3(br_ddot) -> Signal Specification8/1
  Signal Specification/1 -> Buoy's States from UAV/1(ru)
  Signal Specification2/1 -> Buoy's States from UAV/3(ru_ddot)
  Signal Specification1/1 -> theta u4/1, Xb/1
  Buoy's States from UAV/2(rb_dot) -> Signal Specification4/1
  Signal Specification4/1 -> theta u6/1, Xdot_b/1
  Signal Specification5/1 -> Buoy's States from UAV/2(ru_dot)
  Signal Specification6/1 -> Buoy's States from UAV/5(br)
  Signal Specification8/1 -> Buoy's States from UAV/7(br_ddot)
  Signal Specification7/1 -> Buoy's States from UAV/6(br_dot)
  Signal Specification3/1 -> theta u1/1, Xddot_b/1

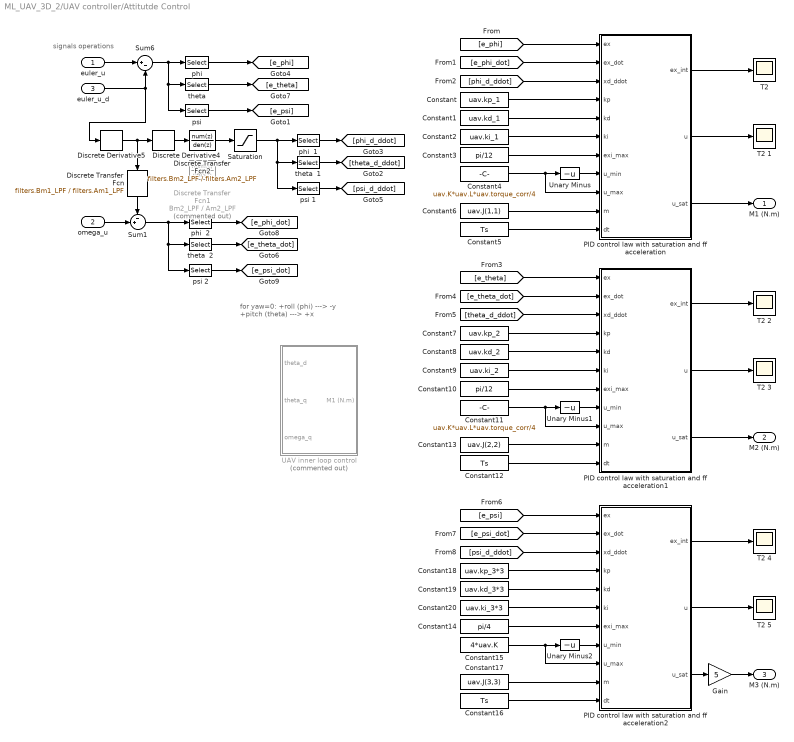
== system ML_UAV_3D_2/UAV controller/Attitutde Control ==
  note: for yaw=0:
      | +roll (phi) ---> -y
      | +pitch (theta) ---> +x
  note: signals operations
  euler_u : Inport
  omega_u : Inport  Port=2
  euler_u_d : Inport  Port=3
  "  phi  " : Selector  InputPortWidth=3  IndexOptions=Index vector (dialog)  Indices=1  OutputSizes=1
  "  phi  1" : Selector  InputPortWidth=3  IndexOptions=Index vector (dialog)  Indices=1  OutputSizes=1
  "  phi  2" : Selector  InputPortWidth=3  IndexOptions=Index vector (dialog)  Indices=1  OutputSizes=1
  "  theta  " : Selector  InputPortWidth=3  IndexOptions=Index vector (dialog)  Indices=2  OutputSizes=1
  "  theta  1" : Selector  InputPortWidth=3  IndexOptions=Index vector (dialog)  Indices=2  OutputSizes=1
  "  theta  2" : Selector  InputPortWidth=3  IndexOptions=Index vector (dialog)  Indices=2  OutputSizes=1
  " psi " : Selector  InputPortWidth=3  IndexOptions=Index vector (dialog)  Indices=3  OutputSizes=1
  " psi 1" : Selector  InputPortWidth=3  IndexOptions=Index vector (dialog)  Indices=3  OutputSizes=1
  " psi 2" : Selector  InputPortWidth=3  IndexOptions=Index vector (dialog)  Indices=3  OutputSizes=1
  Constant : Constant  Value=uav.kp_1
  Constant1 : Constant  Value=uav.kd_1
  Constant10 : Constant  Value=pi/12
  Constant11 : Constant  Value=uav.K*uav.L*uav.torque_corr/4
  Constant12 : Constant  Value=Ts
  Constant13 : Constant  Value=uav.J(2,2)
  Constant14 : Constant  Value=pi/4
  Constant15 : Constant  Value=4*uav.K
  Constant16 : Constant  Value=Ts
  Constant17 : Constant  Value=uav.J(3,3)
  Constant18 : Constant  Value=uav.kp_3*3
  Constant19 : Constant  Value=uav.kd_3*3
  Constant2 : Constant  Value=uav.ki_1
  Constant20 : Constant  Value=uav.ki_3*3
  Constant3 : Constant  Value=pi/12
  Constant4 : Constant  Value=uav.K*uav.L*uav.torque_corr/4
  Constant5 : Constant  Value=Ts
  Constant6 : Constant  Value=uav.J(1,1)
  Constant7 : Constant  Value=uav.kp_2
  Constant8 : Constant  Value=uav.kd_2
  Constant9 : Constant  Value=uav.ki_2
  Discrete Transfer Fcn : DiscreteTransferFcn  Numerator=filters.Bm1_LPF  Denominator=filters.Am1_LPF  InitialStates=[0;0;0]
  Discrete Transfer Fcn1 : DiscreteTransferFcn  Commented=on  Numerator=Bm2_LPF  Denominator=Am2_LPF  InitialStates=[0 0 0]
  Discrete Transfer Fcn2 : DiscreteTransferFcn  Numerator=filters.Bm2_LPF  Denominator=filters.Am2_LPF
  Discrete Derivative4 : simulink/Discrete/Discrete Derivative  gainval=1.0  ICPrevScaledInput=uav.euler_0  OutMin=[]  OutMax=[]  OutDataType=fixdt(1, 16)  OutScaling=2^-10  DoSatur=off
  Discrete Derivative5 : simulink/Discrete/Discrete Derivative  gainval=1.0  ICPrevScaledInput=[uav.euler_0]/Ts  OutMin=[]  OutMax=[]  OutDataType=fixdt(1, 16)  OutScaling=2^-10  DoSatur=off
  Gain : Gain  Gain=5
  PID control law with saturation and ff acceleration : MATLAB Function  TreatAsAtomicUnit=on
  PID control law with saturation and ff acceleration1 : MATLAB Function  TreatAsAtomicUnit=on
  PID control law with saturation and ff acceleration2 : MATLAB Function  TreatAsAtomicUnit=on
  Saturation : Saturate  UpperLimit=[5 5 5]  LowerLimit=-[5 5 5]
  Sum1 : Sum  Inputs=-+|
  Sum6 : Sum  Inputs=|+-
  T2 {,1..5} (6 alike) : Scope
  UAV inner loop control : Subsystem  Commented=on
  Unary Minus : UnaryMinus
  Unary Minus1 : UnaryMinus
  Unary Minus2 : UnaryMinus
  M1 (N.m) : Outport
  M2 (N.m) : Outport  Port=2
  M3 (N.m) : Outport  Port=3
  wires:
  "  phi  "/1 -> [e_phi]
  omega_u/1 -> Sum1/2
  "  theta  "/1 -> [e_theta]
  euler_u_d/1 -> Discrete Derivative5/1, Sum6/2
  Discrete Derivative5/1 -> Discrete Derivative4/1, Discrete Transfer Fcn/1
  Sum6/1 -> " psi "/1, "  theta  "/1, "  phi  "/1
  euler_u/1 -> Sum6/1
  Sum1/1 -> " psi 2"/1, "  theta  2"/1, "  phi  2"/1
  " psi "/1 -> [e_psi]
  Saturation/1 -> "  phi  1"/1, " psi 1"/1, "  theta  1"/1
  "  phi  1"/1 -> [phi_d_ddot]
  "  theta  1"/1 -> [theta_d_ddot]
  " psi 1"/1 -> [psi_d_ddot]
  "  phi  2"/1 -> [e_phi_dot]
  "  theta  2"/1 -> [e_theta_dot]
  " psi 2"/1 -> [e_psi_dot]
  [e_phi_dot] -> PID control law with saturation and ff acceleration/2(ex_dot)
  [e_phi] -> PID control law with saturation and ff acceleration/1(ex)
  [phi_d_ddot] -> PID control law with saturation and ff acceleration/3(xd_ddot)
  Constant/1 -> PID control law with saturation and ff acceleration/4(kp)
  Constant2/1 -> PID control law with saturation and ff acceleration/6(ki)
  Constant1/1 -> PID control law with saturation and ff acceleration/5(kd)
  Constant3/1 -> PID control law with saturation and ff acceleration/7(exi_max)
  Constant4/1 -> PID control law with saturation and ff acceleration/9(u_max), Unary Minus/1
  Unary Minus/1 -> PID control law with saturation and ff acceleration/8(u_min)
  Constant5/1 -> PID control law with saturation and ff acceleration/11(dt)
  Constant6/1 -> PID control law with saturation and ff acceleration/10(m)
  PID control law with saturation and ff acceleration/1(ex_int) -> "T2 "/1
  PID control law with saturation and ff acceleration/2(u) -> T2 1/1
  PID control law with saturation and ff acceleration/3(u_sat) -> M1 (N.m)/1
  PID control law with saturation and ff acceleration1/2(u) -> T2 3/1
  [e_theta_dot] -> PID control law with saturation and ff acceleration1/2(ex_dot)
  Constant13/1 -> PID control law with saturation and ff acceleration1/10(m)
  [e_theta] -> PID control law with saturation and ff acceleration1/1(ex)
  [theta_d_ddot] -> PID control law with saturation and ff acceleration1/3(xd_ddot)
  PID control law with saturation and ff acceleration1/3(u_sat) -> M2 (N.m)/1
  Constant7/1 -> PID control law with saturation and ff acceleration1/4(kp)
  Constant9/1 -> PID control law with saturation and ff acceleration1/6(ki)
  Constant8/1 -> PID control law with saturation and ff acceleration1/5(kd)
  Unary Minus1/1 -> PID control law with saturation and ff acceleration1/8(u_min)
  Constant10/1 -> PID control law with saturation and ff acceleration1/7(exi_max)
  PID control law with saturation and ff acceleration1/1(ex_int) -> T2 2/1
  Constant11/1 -> PID control law with saturation and ff acceleration1/9(u_max), Unary Minus1/1
  Constant12/1 -> PID control law with saturation and ff acceleration1/11(dt)
  PID control law with saturation and ff acceleration2/3(u_sat) -> Gain/1
  Constant14/1 -> PID control law with saturation and ff acceleration2/7(exi_max)
  PID control law with saturation and ff acceleration2/1(ex_int) -> T2 4/1
  Unary Minus2/1 -> PID control law with saturation and ff acceleration2/8(u_min)
  Constant18/1 -> PID control law with saturation and ff acceleration2/4(kp)
  Constant15/1 -> PID control law with saturation and ff acceleration2/9(u_max), Unary Minus2/1
  [e_psi] -> PID control law with saturation and ff acceleration2/1(ex)
  [psi_d_ddot] -> PID control law with saturation and ff acceleration2/3(xd_ddot)
  Constant16/1 -> PID control law with saturation and ff acceleration2/11(dt)
  Constant17/1 -> PID control law with saturation and ff acceleration2/10(m)
  PID control law with saturation and ff acceleration2/2(u) -> T2 5/1
  [e_psi_dot] -> PID control law with saturation and ff acceleration2/2(ex_dot)
  Constant20/1 -> PID control law with saturation and ff acceleration2/6(ki)
  Constant19/1 -> PID control law with saturation and ff acceleration2/5(kd)
  Discrete Derivative4/1 -> Discrete Transfer Fcn2/1
  Discrete Transfer Fcn/1 -> Sum1/1
  Discrete Transfer Fcn2/1 -> Saturation/1
  Gain/1 -> M3 (N.m)/1

== system ML_UAV_3D_2/UAV controller/Decoupling control signals  ==
  Us : Inport
  "alpha, phi" : Inport  Port=2
  psi_u : Inport  Port=3
  Constant1 : Constant  Value=uav.LIMIT_uCMD_HEIGHT
  Constant2 : Constant  Value=uav.LIMIT_CMD_PITCH
  Constant3 : Constant  Value=uav.m*g*0.5
  Demux : Demux  Outputs=3
  Demux1 : Demux  Outputs=2
  U_C{,1..5} (6 alike) : Scope
  control signals decoupling : MATLAB Function  TreatAsAtomicUnit=on
  u1 : Outport
  phi_u : Outport  Port=2
  theta_u : Outport  Port=3
  wires:
  Constant3/1 -> control signals decoupling/7(uz_min)
  Constant1/1 -> control signals decoupling/8(u1_max)
  Constant2/1 -> control signals decoupling/9(tilt_max)
  Demux/2 -> control signals decoupling/2(ua)
  Demux/1 -> control signals decoupling/1(ur)
  Demux/3 -> control signals decoupling/3(uf)
  Us/1 -> U_C4/1, Demux/1
  Demux1/2 -> control signals decoupling/5(phi)
  Demux1/1 -> control signals decoupling/4(alpha)
  psi_u/1 -> control signals decoupling/6(psi_u)
  control signals decoupling/4(theta_u) -> U_C3/1, theta_u/1
  control signals decoupling/1(u_C) -> U_C/1
  control signals decoupling/2(u1) -> U_C1/1, u1/1
  control signals decoupling/3(phi_u) -> U_C2/1, phi_u/1
  "alpha, phi"/1 -> U_C5/1, Demux1/1

== system ML_UAV_3D_2/UAV controller/Enabled Subsystem1 ==
  u : Inport
  reset : Inport  Port=2
  u0 : Inport  Port=3
  Enable : EnablePort
  Logical Operator : Logic  Operator=NOT  AllPortsSameDT=off  OutDataTypeStr=boolean
  Low Pass Filter5 : DiscreteTransferFcn  Numerator=filters.Bm_rdeL_LPF  Denominator=filters.Am_rdeL_LPF  InitialStatesSource=Input port  ExternalReset=Level
      settings: InputPortMap=u0,r7,p5
  Mux2 : Mux  Inputs=2
  adjustment for this specific transfer function : Gain  Gain=84.6505602
  r_dot filt : Scope
  r_dot filt1 : Scope
  y : Outport
  wires:
  u/1 -> Mux2/2, Low Pass Filter5/1
  Low Pass Filter5/1 -> Mux2/1, y/1
  Logical Operator/1 -> r_dot filt1/1, Low Pass Filter5/2
  u0/1 -> adjustment for this specific transfer function/1
  Mux2/1 -> r_dot filt/1
  adjustment for this specific transfer function/1 -> Low Pass Filter5/3
  reset/1 -> Logical Operator/1

== system ML_UAV_3D_2/UAV controller/cond1 ==
  r : Inport
  r_dot : Inport  Port=2
  coupled : Inport  Port=3
  Constant : Constant  Value=cable.L_0
  Constant2 : Constant  Value=Ts
  MATLAB Function : MATLAB Function  TreatAsAtomicUnit=on
  r_dot filt2 : Scope
  key : Outport
  wires:
  r/1 -> MATLAB Function/1(r)
  Constant/1 -> MATLAB Function/4(Lc)
  Constant2/1 -> MATLAB Function/5(dt)
  MATLAB Function/1(y) -> key/1
  r_dot/1 -> MATLAB Function/2(r_dot)
  coupled/1 -> MATLAB Function/3(coupled)
  MATLAB Function/2(t) -> r_dot filt2/1

== system ML_UAV_3D_2/UAV controller/rdot 0 ==
  X : Inport
  Trigger : TriggerPort  VariantControl=Variant
  Xu_init : Outport
  wires:
  X/1 -> Xu_init/1
